simulink model "main_direct"  (R2022b)
settings: Solver=ode45  StartTime=0.0  StopTime=10  RelTol=1e-3  EnableMultiTasking=on
InitFcn:
  | clear functions
  | % initialize
  | 
  | m = 5;       % total mass (kg)
  | g = 9.8;     % gravitational constant (m/s^2)
  | Ix = 10;     % moment of Inertia (N/m)
  | Iy = 10;
  | Iz = 10;
  | A_qc = [ 0. ,  1. ,  0. ,  0. ,  0. ,  0. ,  0. ,  0. ,  0. ,  0. ,  0. , 0. ;
  |          0. ,  0. ,  0. ,  0. ,  0. ,  0. ,  0. ,  0. ,  0. ,  0. ,  0. , 0. ;
  |          0. ,  0. ,  0. ,  1. ,  0. ,  0. ,  0. ,  0. ,  0. ,  0. ,  0. , 0. ;
  |          0. ,  0. ,  0. ,  0. ,  0. ,  0. ,  0. ,  0. ,  0. ,  0. ,  0. , 0. ;
  |          0. ,  0. ,  0. ,  0. ,  0. ,  1. ,  0. ,  0. ,  0. ,  0. ,  0. , 0. ;
  |          0. ,  0. ,  0. ,  0. ,  0. ,  0. ,  g,  0. ,  0. ,  0. ,  0. , 0. ;
  |          0. ,  0. ,  0. ,  0. ,  0. ,  0. ,  0. ,  1. ,  0. ,  0. ,  0. , 0. ;
  |          0. ,  0. ,  0. ,  0. ,  0. ,  0. ,  0. ,  0. ,  0. ,  0. ,  0. , 0. ;
  |          0. ,  0. ,  0. ,  0. ,  0. ,  0. ,  0. ,  0. ,  0. ,  1. ,  0. , 0. ;
  |          0. ,  0. ,  0. ,  0. ,  0. ,  0. ,  0. ,  0. ,  0. ,  0. , -g, 0. ;
  |          0. ,  0. ,  0. ,  0. ,  0. ,  0. ,  0. ,  0. ,  0. ,  0. ,  0. , 1. ;
  |          0. ,  0. ,  0. ,  0. ,  0. ,  0. ,  0. ,  0. ,  0. ,  0. ,  0. , 0. ];
  | B_qc = zeros(12,4);
  | B_qc(2, 1) = 1 / m;
  | B_qc(4, 2) = 1 / Ix;
  | B_qc(8, 3) = 1 / Iy;
  | B_qc(12, 4) = 1 / Iz;
  | C_qc = eye(12);
  | C1_qc = zeros(4,12);
  | C1_qc(1,1)=1;
  | C1_qc(2,2)=1;
  | C1_qc(3,3)=1;
  | C1_qc(4,4)=1;
  | C2_qc = zeros(8,12);
  | C2_qc(1,5)=1;
  | C2_qc(2,6)=1;
  | C2_qc(3,7)=1;
  | C2_qc(4,8)=1;
  | C2_qc(5,9)=1;
  | C2_qc(6,10)=1;
  | C2_qc(7,11)=1;
  | C2_qc(8,12)=1;
  | D_qc = zeros(size(C_qc,1), size(B_qc,2));
  | D1_qc = zeros(size(C1_qc,1), size(B_qc,2));
  | D2_qc = zeros(size(C2_qc,1), size(B_qc,2));
  | KK = [3.12685594967393	5.60056530879117	-8.20209119000962e-15	-1.04128354000384e-13	-1.98079971800411e-12	-2.80542422407473e-12	-1.99114681683400e-11	-7.24706879962799e-12	-1.39173410223583e-13	-3.33838482828459e-13	4.33507358703653e-12	2.95847517281528e-12;
  | -2.27958236698399e-15	-5.25758397334492e-14	0.315427247946649	2.53141053716782	2.99704496279930e-13	4.74063575809426e-13	3.84107318902310e-12	1.70079220563172e-12	2.52299350682869e-13	3.76745833724641e-13	-2.98090673411387e-12	-1.26797972193613e-12;
  | -1.93677340409378e-12	-3.55364590767484e-12	3.37102893941443e-13	1.67605514791903e-12	3.05441194111679	6.05997082436238	58.7631166321155	34.1120666564246	5.26929014784828e-12	-4.88953537034324e-12	1.11815184366346e-10	5.76894498698533e-11;
  | 2.22959220224651e-12	1.47614324499605e-12	-4.58040227906012e-13	-1.24705734681365e-12	-2.93867785501474e-11	-2.19347204056775e-11	-1.47234091605739e-11	5.66269232222735e-11	-3.05441194117077	-6.05997082447233	58.7631166330827	34.1120666568239];
  | KK_8 = [3.14806101403323	5.61958299359191	-1.06574271596490e-13	-3.51167300129546e-13	1.41342271329799e-12	2.01062101868168e-12	1.01336113292644e-11	2.21595181457621e-11	-6.09240741105249e-14	5.22728093268344e-16	-2.29214005150142e-13	-1.63828525072864e-14
  | -1.40612070043267e-13	-1.55665450866325e-13	0.315907315209643	2.53336608803131	6.85283776603311e-13	8.93097231937326e-13	5.64678083994045e-12	1.85029586289379e-12	2.38846862222207e-13	3.94653870911855e-13	-2.69539769628066e-12	-1.50278419750555e-12
  | 6.06951163104689e-12	1.09751533138976e-11	1.16215441377720e-13	1.84009321132151e-12	3.11868152834707	6.16850483139175	59.6311710091072	34.4660711180138	4.69926930228626e-11	7.26917658867268e-11	-5.24662404659150e-10	-1.89171664196777e-10
  | 4.93997661255683e-13	-7.79648124187351e-15	-3.11282929182986e-13	-1.50718804881790e-12	-5.37309119167142e-11	-7.78148637957717e-11	-5.41596347348106e-10	-1.89400019326547e-10	-3.11868152830212	-6.16850483132701	59.6311710086223	34.4660711178274];
  | 
  | Q_qc = diag([100, 1, 1, 1, 100, 1, 1, 1, 100, 1, 1, 1]);
  | R_qc = diag([10, 10, 10, 10]);
values from neighbouring files (symbols this model uses):
  A_cc = [0 1 0 ... (first row only)    [initialize.m]    (also in initialize2.m)
  A_esp = [-16.95,  -2.365 ... (first row only)    [initialize.m]    (also in initialize2.m)
  A_sc = [3.957e-14  1  1.351e-14   1.193e-16 ... (first row only)    [initialize.m]    (also in initialize2.m)
  A_ttc = [0,1;0,0]    [initialize.m]    (also in initialize2.m)
  B_cc = [0; 0; 2.4767]    [initialize.m]    (also in initialize2.m)
  B_esp = [8.478 ... (first row only)    [initialize.m]    (also in initialize2.m)
  B_sc = [9.628e-15; 80; 20; -1120]    [initialize.m]    (also in initialize2.m)
  B_ttc = [0;1]    [initialize.m]    (also in initialize2.m)
  C_cc = [1 0 0]    [initialize.m]    (also in initialize2.m)
  C_esp = [0,1]    [initialize.m]    (also in initialize2.m)
  C_sc = [1 0 0 0]    [initialize.m]    (also in initialize2.m)
  C_ttc = [1,0]    [initialize.m]    (also in initialize2.m)
  D_cc = [0]    [initialize.m]    (also in initialize2.m)
  D_esp = [0]    [initialize.m]    (also in initialize2.m)
  D_sc = [0]    [initialize.m]    (also in initialize2.m)
  D_ttc = [0]    [initialize.m]    (also in initialize2.m)
undefined symbols (not defined in the file or in its folder): sharedmem
libraries: truetime x1
settings Model: Creator=anton  LastModifiedBy=sunan
settings SolverCC: AlgebraicLoopSolver=TrustRegion
settings DataIOCC: SaveFormat=Array  SignalLoggingSaveFormat=ModelDataLogs  ReturnWorkspaceOutputs=off
settings OptimizationCC: BlockReduction=off  BooleanDataType=off  ExpressionDepthLimit=2147483647  LifeSpan=inf
settings DebuggingCC: SaveWithParameterizedLinksMsg=none  UnderspecifiedInitializationDetection=Classic  MergeDetectMultiDrivingBlocksExec=none  SignalResolutionControl=TryResolveAllWithWarning  MultiTaskDSMMsg=warning  MultiTaskCondExecSysMsg=none  FcnCallInpInsideContextMsg=warning  UnconnectedInputMsg=warning  UnconnectedOutputMsg=warning  UnconnectedLineMsg=warning  StateNameClashWarn=warning  SFUnexpectedBacktrackingDiag=warning  SFNoUnconditionalDefaultTransitionDiag=warning  SFExecutionAtInitializationDiag=none  SFMachineParentedDataDiag=warning  ArithmeticOperatorsInVariantConditions=warning
settings HardwareCC: ProdBitPerPointer=32  ProdBitPerSizeT=32  ProdBitPerPtrDiffT=32  ProdLargestAtomicFloat=None  ProdIntDivRoundTo=Undefined  ProdEndianess=Unspecified  ProdWordSize=32  ProdHWDeviceType=32-bit Generic  TargetUnknown=on
settings ModelReferenceCC: EnableRefExpFcnMdlSchedulingChecks=on  PropagateSignalLabelsOutOfModel=off
settings SFSimCC: SimUseLocalCustomCode=off  CustomCodeUndefinedFunction=UseInterfaceOnly
settings RTWCC: RTWUseLocalCustomCode=off  DLArmComputeVersion=19.05
settings CodeAppCC: StateflowObjectComments=on
settings GRTTargetCC: TargetLangStandard=C89/C90 (ANSI)  CombineOutputUpdateFcns=off  GRTInterface=on
settings ConfigComp: CovMetricSettings=dw  CovSaveCumulativeToWorkspaceVar=on  CovSaveSingleToWorkspaceVar=on  CovExternalEMLEnable=off

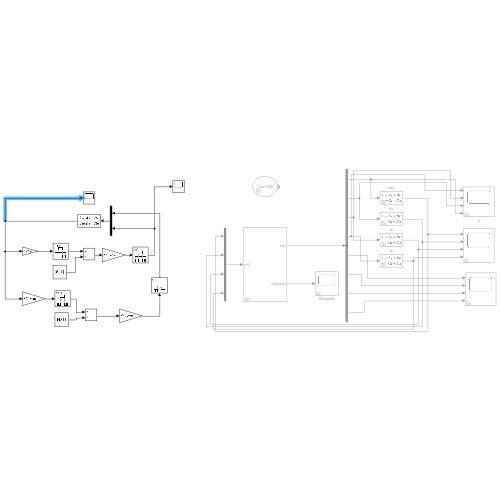
[thumbnail: Simulink's stored preview of the top-level diagram]
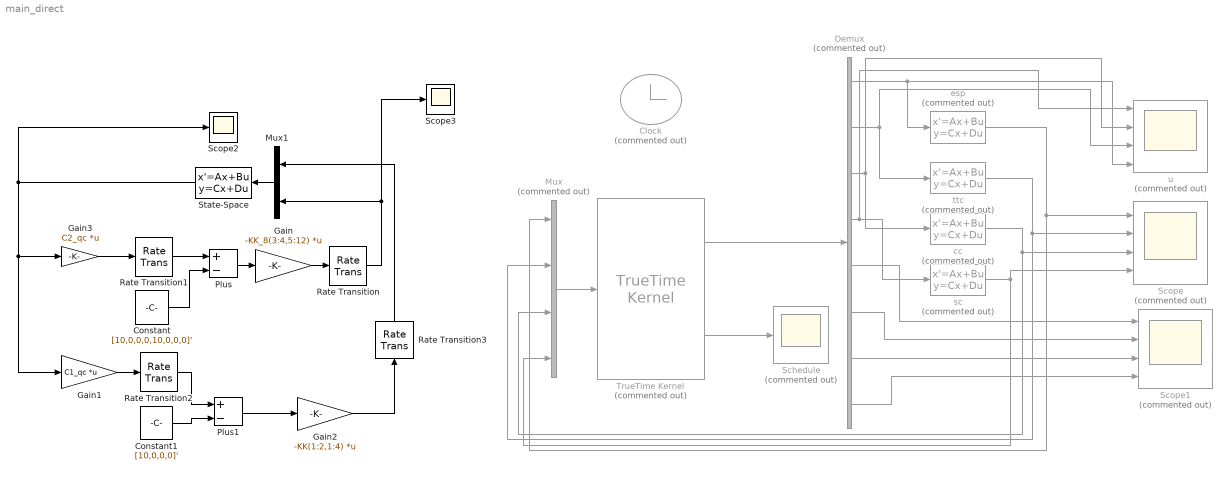
== system main_direct ==
  Clock : Clock  Commented=on
  Constant : Constant  Value=[10,0,0,0,10,0,0,0]'  SampleTime=0.02
  Constant1 : Constant  Value=[10,0,0,0]'  SampleTime=0.02
  Demux : Demux  Commented=on  Outputs=8
      settings: DisplayOption=none
  Gain : Gain  Gain=-KK_8(3:4,5:12)  Multiplication=Matrix(K*u) (u vector)
  Gain1 : Gain  Gain=C1_qc  Multiplication=Matrix(K*u) (u vector)
  Gain2 : Gain  Gain=-KK(1:2,1:4)  Multiplication=Matrix(K*u) (u vector)
  Gain3 : Gain  Gain=C2_qc  Multiplication=Matrix(K*u) (u vector)
  Mux : Mux  Commented=on
  Mux1 : Mux  Inputs=2
  Plus : Sum  Inputs=+-
  Plus1 : Sum  Inputs=+-
  Rate Transition : RateTransition  InitialCondition=zeros(2,1)
  Rate Transition1 : RateTransition  InitialCondition=zeros(8,1)  OutPortSampleTime=0.008
  Rate Transition2 : RateTransition  InitialCondition=zeros(4,1)  OutPortSampleTime=0.02
  Rate Transition3 : RateTransition  InitialCondition=zeros(2,1)
  Schedule : Scope  Commented=on
  Scope : Scope  Commented=on  NumInputPorts=4
  Scope1 : Scope  Commented=on  NumInputPorts=4
  Scope2 : Scope
  Scope3 : Scope
  State-Space : StateSpace  A=A_qc  B=B_qc  C=C_qc  D=D_qc  InitialCondition=zeros(12,1)
  TrueTime Kernel : truetime/TrueTime Kernel  Commented=on  sfun=control_sched_init  args=Systems  ninputsoutputs=[4 8]  ntriggers=0  trigtype=falling  nwnodenbr=[]  clockoffsetdrift=[0 0]  schedoutput=on  battery=off  poweroutput=off
  cc : StateSpace  Commented=on  A=A_cc  B=B_cc  C=C_cc  D=D_cc  InitialCondition=sharedmem.x0{3}
  esp : StateSpace  Commented=on  A=A_esp  B=B_esp  C=C_esp  D=D_esp  InitialCondition=sharedmem.x0{1}
  sc : StateSpace  Commented=on  A=A_sc  B=B_sc  C=C_sc  D=D_sc  InitialCondition=sharedmem.x0{4}
  ttc : StateSpace  Commented=on  A=A_ttc  B=B_ttc  C=C_ttc  D=D_ttc  InitialCondition=sharedmem.x0{2}
  u : Scope  Commented=on  NumInputPorts=4
  wires:
  esp/1 -> Mux/1, Scope/1
  sc/1 -> Scope/4, Mux/4
  Mux/1 -> TrueTime Kernel/1
  TrueTime Kernel/1 -> Demux/1
  cc/1 -> Mux/3, Scope/3
  ttc/1 -> Mux/2, Scope/2
  TrueTime Kernel/2 -> Schedule/1
  Demux/4 -> sc/1, u/1
  Demux/3 -> cc/1, u/2
  Demux/2 -> ttc/1, u/3
  Demux/1 -> esp/1, u/4
  Demux/5 -> Scope1/1
  Demux/6 -> Scope1/2
  Demux/7 -> Scope1/3
  Demux/8 -> Scope1/4
  Gain/1 -> Rate Transition/1
  Rate Transition1/1 -> Plus/1
  Constant/1 -> Plus/2
  Plus/1 -> Gain/1
  Gain1/1 -> Rate Transition2/1
  Rate Transition2/1 -> Plus1/1
  Constant1/1 -> Plus1/2
  State-Space/1 -> Scope2/1, Gain3/1, Gain1/1
  Plus1/1 -> Gain2/1
  Gain2/1 -> Rate Transition3/1
  Rate Transition/1 -> Scope3/1, Mux1/2
  Rate Transition3/1 -> Mux1/1
  Mux1/1 -> State-Space/1
  Gain3/1 -> Rate Transition1/1
